simulink model "LQR_Controller"  (R2025a)
settings: Solver=FixedStepDiscrete  StartTime=0.0  StopTime=Inf  FixedStep=0.0035  RelTol=1e-3  EnableMultiTasking=on
model workspace (MAT data in the model file):
  R_motor = 6
  encoderDt = 0.014
  k_motor = 0.076
  r = 0.0065
undefined symbols (not defined in the file or in its folder): DiscIntNeverNeededParam
libraries: arduinolib x5, dspstat3 x2, simulink x1, arduinosensorlib x1
settings Model: SimulationMode=external  SILPILModeSetting=veronly  ExtModeTrigDuration=2  Creator=Hudso  LastModifiedBy=Hudso
settings SolverCC: AutoInsertRateTranBlk=on
settings OptimizationCC: EnhancedBackFolding=on  PassReuseOutputArgsAs=Individual arguments  ZeroExternalMemoryAtStartup=off  ZeroInternalMemoryAtStartup=off  MaxStackSize=64  OptimizeBlockOrder=speed  DifferentSizesBufferReuse=on  OptimizationCustomize=off  EfficientTunableParamExpr=on
settings DebuggingCC: ParamPrecisionLossAbsoluteDiffThreshold=1e-4  ParamPrecisionLossRelativeDiffThreshold=1e-4  ParameterTunabilityLossMsg=error
settings HardwareCC: ProdBitPerInt=16.0  ProdBitPerPointer=16.0  ProdBitPerSizeT=16.0  ProdBitPerPtrDiffT=16.0  ProdLargestAtomicFloat=None  ProdWordSize=8.0  ProdLongLongMode=on  ProdHWDeviceType=Atmel->AVR  UseEmbeddedCoderFeatures=off
settings SFSimCC: MATLABDynamicMemAlloc=off
settings RTWCC: SystemTargetFile=ert.tlc  HardwareBoard=Arduino Uno  TemplateMakefile=ert_default_tmf  Toolchain=Arduino AVR  BuildConfiguration=Faster Runs  Description=Embedded Coder
settings CodeAppCC: ForceParamTrailComments=on  IgnoreCustomStorageClasses=off  OperatorAnnotations=on  SimulinkDataObjDesc=on  SFDataObjDesc=on  InsertBlockDesc=on
settings ERTTargetCC: ExtModeTransport=3.0  ExtModeAutomaticAllocSize=off  ExtModeStaticAllocSize=250.0  InlinedParameterPlacement=Hierarchical  SupportContinuousTime=on  SupportNonInlinedSFcns=on  SupportVariableSizeSignals=on

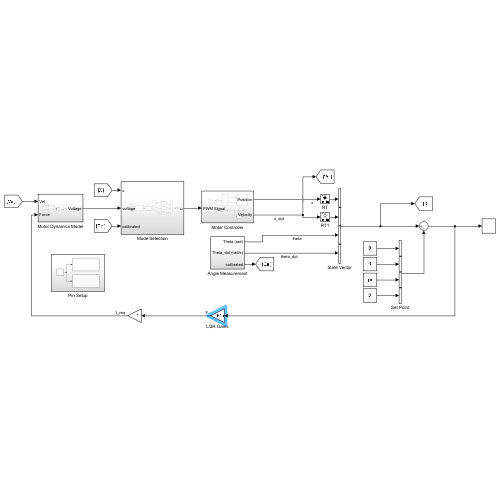
[thumbnail: Simulink's stored preview of the top-level diagram]
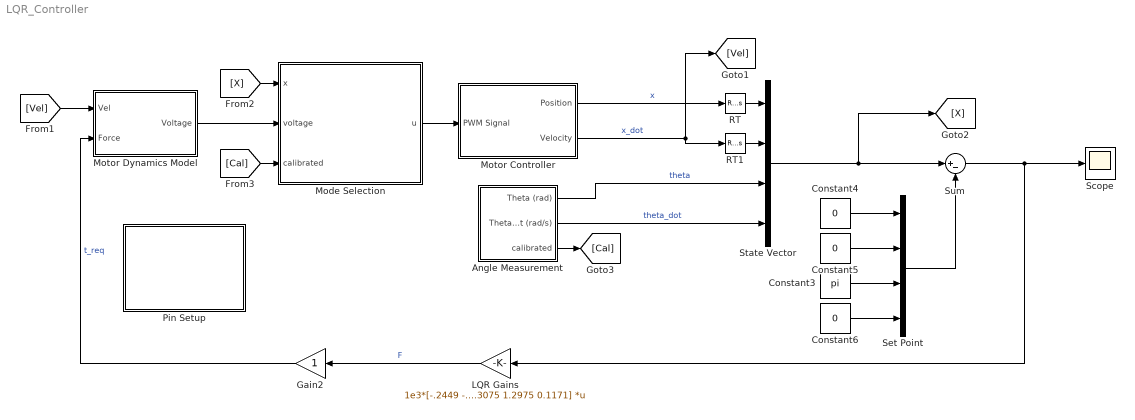
== system LQR_Controller ==
  Angle Measurement : Subsystem
  Constant3 : Constant  Value=pi
  Constant4 : Constant  Value=0
  Constant5 : Constant  Value=0
  Constant6 : Constant  Value=0
  Gain2 : Gain
  LQR Gains : Gain  Gain=1e3*[-.2449 -.3075 1.2975 0.1171]  Multiplication=Matrix(K*u)
  Mode Selection : Subsystem
  Motor Controller : Subsystem
  Motor Dynamics Model : Subsystem
  Pin Setup : Subsystem
  RT : RateTransition
  RT1 : RateTransition  OutPortSampleTime=0.007
  Scope : Scope
      settings: ActiveDisplayYMinimum=-0.46421626351926437  ActiveDisplayYMaximum=0.39329876424662991
  Set Point : Concatenate  NumInputs=4
  State Vector : Concatenate  NumInputs=4
  Sum : Sum  Inputs=|+-
  wires:
  Angle Measurement/1(Theta (rad)) -> State Vector/3  "theta"
  Motor Controller/1(Position) -> RT/1  "x"
  Motor Controller/2(Velocity) -> [Vel], RT1/1  "x_dot"
  Angle Measurement/2(Theta_dot (rad/s)) -> State Vector/4  "theta_dot"
  LQR Gains/1 -> Gain2/1  "F"
  Constant3/1 -> Set Point/3
  Constant4/1 -> Set Point/1
  Constant5/1 -> Set Point/2
  Constant6/1 -> Set Point/4
  State Vector/1 -> [X], Sum/1
  Sum/1 -> Scope/1, LQR Gains/1
  Set Point/1 -> Sum/2
  [Vel] -> Motor Dynamics Model/1(Vel)
  Gain2/1 -> Motor Dynamics Model/2(Force)  "t_req"
  RT/1 -> State Vector/1
  RT1/1 -> State Vector/2
  Angle Measurement/3(calibrated) -> [Cal]
  [X] -> Mode Selection/1(x)
  [Cal] -> Mode Selection/3(calibrated)
  Mode Selection/1(u) -> Motor Controller/1(PWM Signal)
  Motor Dynamics Model/1(Voltage) -> Mode Selection/2(voltage)

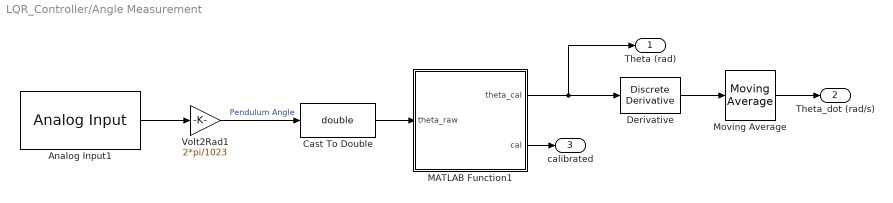
== system LQR_Controller/Angle Measurement ==
  Analog Input1 : arduinolib/Analog Input  pinNumber=0  ReadResultsOnly=off  ConversionTriggerSource=Software  ExternalTriggerType=uint32( 0 )  OutputDataType=uint16  EnableConversionCompleteNotify=off  EnableOuputStatus=off  SampleTime=-1  blockPlatform=arduino
  Cast To Double : DataTypeConversion  OutDataTypeStr=double  SaturateOnIntegerOverflow=off  RndMeth=Floor
  Derivative : simulink/Discrete/Discrete Derivative  gainval=1.0  ICPrevScaledInput=0.0  OutMin=[]  OutMax=[]  OutDataType=fixdt(1, 16)  OutScaling=2^-10  RndMeth=Nearest  DoSatur=off
  MATLAB Function1 : MATLAB Function  TreatAsAtomicUnit=on
  Moving Average : dspstat3/Moving Average  Method=Sliding window  ForgettingFactorPort=off  SpecifyWindowLength=on  WindowLength=12  OverlapLength=11  AllowArbitraryInputLength=off  ForgettingFactor=0.9  SimulateUsing=Interpreted execution
  Volt2Rad1 : Gain  Gain=2*pi/1023
  Theta (rad) : Outport
  Theta_dot (rad/s) : Outport  Port=2
  calibrated : Outport  Port=3
  wires:
  Analog Input1/1 -> Volt2Rad1/1
  Volt2Rad1/1 -> Cast To Double/1  "Pendulum Angle"
  Cast To Double/1 -> MATLAB Function1/1(theta_raw)
  MATLAB Function1/1(theta_cal) -> Derivative/1, Theta (rad)/1
  Derivative/1 -> Moving Average/1
  Moving Average/1 -> Theta_dot (rad/s)/1
  MATLAB Function1/2(cal) -> calibrated/1

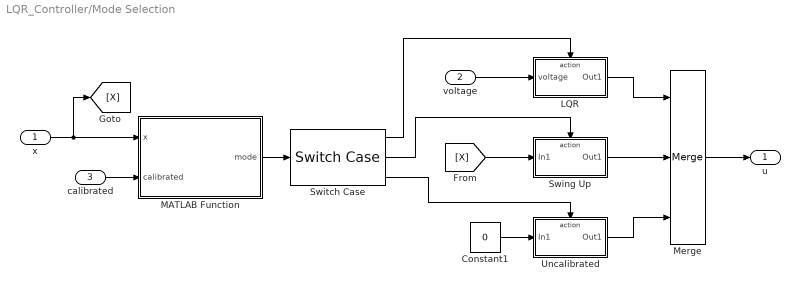
== system LQR_Controller/Mode Selection ==
  x : Inport
  voltage : Inport  Port=2
  calibrated : Inport  Port=3
  Constant1 : Constant  Value=0
  LQR : Subsystem  TreatAsAtomicUnit=on
  MATLAB Function : MATLAB Function  TreatAsAtomicUnit=on
  Merge : Merge  Inputs=3
  Swing Up : Subsystem  TreatAsAtomicUnit=on
  Switch Case : SwitchCase  CaseConditions={1,2}
  Uncalibrated : Subsystem  TreatAsAtomicUnit=on
  u : Outport
  wires:
  calibrated/1 -> MATLAB Function/2(calibrated)
  x/1 -> [X], MATLAB Function/1(x)
  MATLAB Function/1(mode) -> Switch Case/1
  Switch Case/1 -> LQR/Action
  LQR/1(Out1) -> Merge/1
  voltage/1 -> LQR/1(voltage)
  Switch Case/2 -> Swing Up/Action
  Swing Up/1(Out1) -> Merge/2
  Merge/1 -> u/1
  Switch Case/3 -> Uncalibrated/Action
  Constant1/1 -> Uncalibrated/1(In1)
  Uncalibrated/1(Out1) -> Merge/3
  [X] -> Swing Up/1(In1)

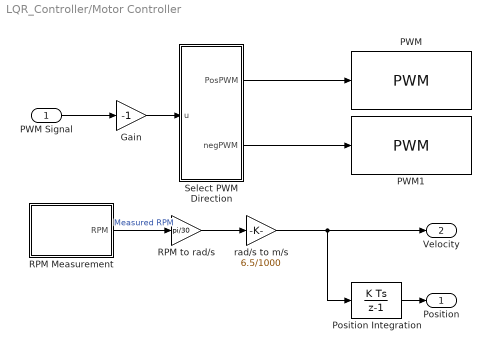
== system LQR_Controller/Motor Controller ==
  PWM Signal : Inport
  Gain : Gain  Gain=-1
  PWM : arduinolib/PWM  pinNumber=5  frequencyType=Default  desiredFrequency=490.2  achievableFrequency=490.2
  PWM1 : arduinolib/PWM  pinNumber=6  frequencyType=Default  desiredFrequency=490.2  achievableFrequency=490.2
  Position Integration : DiscreteIntegrator  SampleTime=encoderDt  LimitOutput=on  UpperSaturationLimit=.5  LowerSaturationLimit=-.5  ICPrevOutput=DiscIntNeverNeededParam  ICPrevScaledInput=DiscIntNeverNeededParam
  RPM Measurement : Subsystem
  RPM to rad/s : Gain  Gain=pi/30
  Select PWM Direction : MATLAB Function  TreatAsAtomicUnit=on
  rad/s to m/s : Gain  Gain=6.5/1000
  Position : Outport
  Velocity : Outport  Port=2
  wires:
  RPM to rad/s/1 -> rad/s to m/s/1
  Select PWM Direction/2(negPWM) -> PWM1/1
  RPM Measurement/1(RPM) -> RPM to rad/s/1  "Measured RPM"
  Position Integration/1 -> Position/1
  Select PWM Direction/1(PosPWM) -> PWM/1
  rad/s to m/s/1 -> Position Integration/1, Velocity/1
  PWM Signal/1 -> Gain/1
  Gain/1 -> Select PWM Direction/1(u)

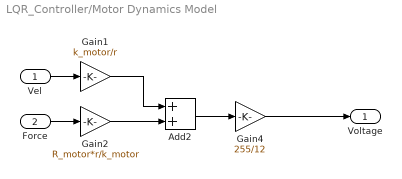
== system LQR_Controller/Motor Dynamics Model ==
  Vel : Inport
  Force : Inport  Port=2
  Add2 : Sum
  Gain1 : Gain  Gain=k_motor/r
  Gain2 : Gain  Gain=R_motor*r/k_motor
  Gain4 : Gain  Gain=255/12
  Voltage : Outport
  wires:
  Gain2/1 -> Add2/2
  Force/1 -> Gain2/1
  Gain1/1 -> Add2/1
  Add2/1 -> Gain4/1
  Gain4/1 -> Voltage/1
  Vel/1 -> Gain1/1

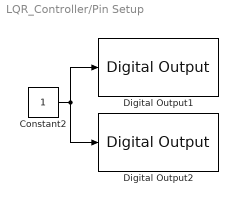
== system LQR_Controller/Pin Setup ==
  Constant2 : Constant
  Digital Output1 : arduinolib/Digital Output  pinNumber=7  Direction=output  blockPlatform=arduino
  Digital Output2 : arduinolib/Digital Output  pinNumber=8  Direction=output  blockPlatform=arduino
  wires:
  Constant2/1 -> Digital Output1/1, Digital Output2/1

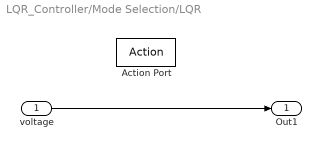
== system LQR_Controller/Mode Selection/LQR ==
  voltage : Inport
  Action Port : ActionPort  ActionPortLabel=case [ 1 ]:
  Out1 : Outport
  wires:
  voltage/1 -> Out1/1

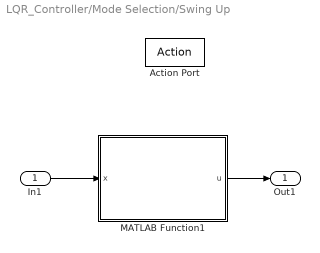
== system LQR_Controller/Mode Selection/Swing Up ==
  In1 : Inport
  Action Port : ActionPort  ActionPortLabel=case [ 2 ]:
  MATLAB Function1 : MATLAB Function  TreatAsAtomicUnit=on
  Out1 : Outport
  wires:
  In1/1 -> MATLAB Function1/1(x)
  MATLAB Function1/1(u) -> Out1/1

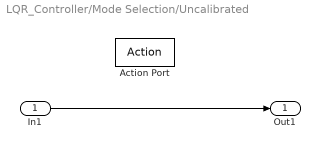
== system LQR_Controller/Mode Selection/Uncalibrated ==
  In1 : Inport
  Action Port : ActionPort  ActionPortLabel=default:
  Out1 : Outport
  wires:
  In1/1 -> Out1/1

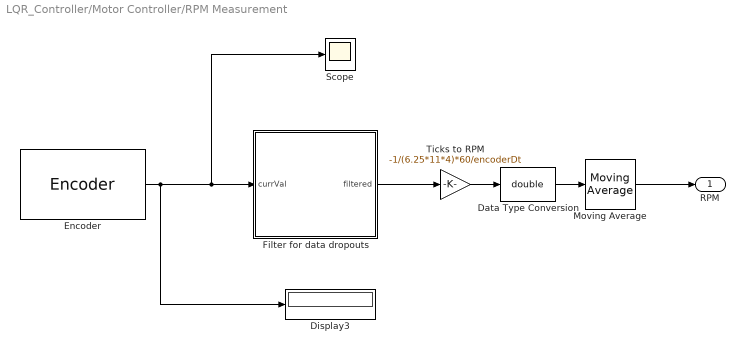
== system LQR_Controller/Motor Controller/RPM Measurement ==
  Data Type Conversion : DataTypeConversion  OutDataTypeStr=double  SaturateOnIntegerOverflow=off  RndMeth=Floor
  Display3 : Display
  Encoder : arduinosensorlib/Encoder  InputA=2  InputB=3  Mode=Reset at each Sample time  SampleTime=encoderDt
  Filter for data dropouts : MATLAB Function  TreatAsAtomicUnit=on
  Moving Average : dspstat3/Moving Average  Method=Sliding window  ForgettingFactorPort=off  SpecifyWindowLength=on  WindowLength=4  OverlapLength=3  AllowArbitraryInputLength=off  ForgettingFactor=0.9  SimulateUsing=Interpreted execution
  Scope : Scope
      settings: ActiveDisplayYMinimum=-1.1468838574999997E+8  ActiveDisplayYMaximum=1.03219438175E+9
  Ticks to RPM : Gain  Gain=-1/(6.25*11*4)*60/encoderDt
  RPM : Outport
  wires:
  Filter for data dropouts/1(filtered) -> Ticks to RPM/1
  Encoder/1 -> Display3/1, Scope/1, Filter for data dropouts/1(currVal)
  Ticks to RPM/1 -> Data Type Conversion/1
  Data Type Conversion/1 -> Moving Average/1
  Moving Average/1 -> RPM/1

== matlab function LQR_Controller/Motor Controller/Select PWM Direction ==
  data: u input; PosPWM output; negPWM output
function [PosPWM, negPWM] = PWMDir(u)
    if u > 0
        PosPWM = u;
        negPWM = 0;
    else
        negPWM = -u;
        PosPWM = 0;
    end
end

== matlab function LQR_Controller/Motor Controller/RPM Measurement/Filter for data dropouts ==
  data: currVal input; filtered output
function filtered = filterEncoder(currVal)
%#codegen

persistent prevVal

% Initialize on first call
if isempty(prevVal)
    prevVal = currVal;
end

% Dropout detection
threshold = 200;  % Adjust based on your system

if abs(currVal - prevVal) > threshold
    % Bad reading: keep previous good value
    filtered = prevVal;
elseif abs(currVal) > 500
    % this is also a bad reading, nothing should be greater than this
    filtered = prevVal;
else
    % Good reading: update and pass through
    filtered = currVal;
    prevVal = currVal;
end

== matlab function LQR_Controller/Mode Selection/MATLAB Function ==
  data: x input; mode output; calibrated input
function mode = ControllerMode(x, calibrated)
% the controller mode selection acts on the state of the pendulum. In the
% standard stable configuration, the controller will center and perform a
% swing up. Once this is achieved, the controller moves into the LQR
% regulator for upright control.
%
% Inputs:
% x - full state vector [4x1]
% voltage - voltage control input [V]
% calibrated - calibration flag boolean

% demux the input state:

pos = x(1);
vel = x(2);
theta = x(3);
omega = x(4);

% if it's calibrated, continue
if calibrated
    % If it is close enough to the vertical position, run the LQR
    if abs(theta-pi) < 0.15 && abs(omega) < 1.5
        mode = 1;        
    else % if it is close enough to the downward position, run the swing up controller
        mode = 2;
    end
else
    mode = 3;
end

end

== matlab function LQR_Controller/Angle Measurement/MATLAB Function1 ==
  data: theta_raw input; theta_cal output; cal output
function [theta_cal, cal] = calibrateAngle(theta_raw)
% Calibrates angle by averaging first N samples at startup,
% then subtracting the average offset and adding pi.
%
% Inputs:
%  - theta_raw : current raw angle measurement
%  - reset     : boolean flag to reset calibration (true at startup)
%
% Output:
%  - theta_cal : calibrated angle (aligned so initial avg = pi)

    persistent sample_count theta_sum theta0 calibrated N

    if isempty(calibrated)
        % Initialization on reset
        N = 250;                % number of samples to average
        sample_count = 0;
        theta_sum = 0;
        theta0 = 0;
        calibrated = false;
        cal = false;
    end

    if ~calibrated
        % Accumulate samples for averaging
        sample_count = sample_count + 1;
        theta_sum = theta_sum + theta_raw;
        
        if sample_count >= N
            theta0 = theta_sum / N;  % average offset
            calibrated = true;
            cal = true;
        end
    end

    if calibrated
        % After calibration, subtract offset and add pi
        theta_cal = theta_raw - theta0 + 2*pi;
        cal = true;
    else
        % During calibration phase, output raw angle
        theta_cal = theta_raw + 1/2*pi; 
        cal = false;
    end
end

== matlab function LQR_Controller/Mode Selection/Swing Up/MATLAB Function1 ==
  data: x input; u output
function u = SwingUpController(x)

% demux the input state:
pos = x(1);
vel = x(2);
theta = x(3);
omega = x(4);

persistent thetaMax

if isempty(thetaMax)
    thetaMax = theta;
end

T = 1.1; % period of pendulum
t = 0.05; % acceleration time of pendulum

alphaBest = thetaMax * sin(2*pi/T*t);

u = 0;

end
